simulink subsystem "evitaparedes"  (R2023b)
settings: Solver=VariableStepAuto  StartTime=0.0  StopTime=10.0  RelTol=1e-3
settings Model: Creator=Usuario_UMA  LastModifiedBy=Usuario_UMA

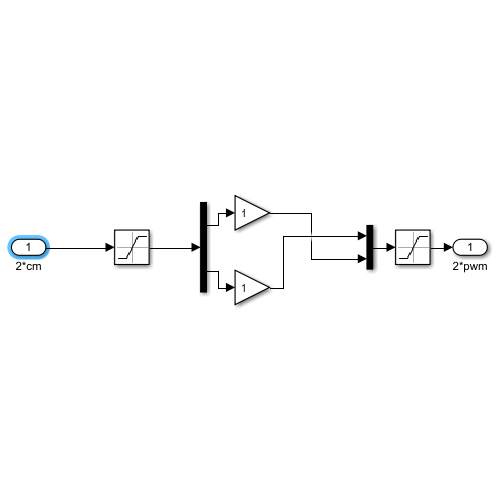
[thumbnail: Simulink's stored preview of the top-level diagram]
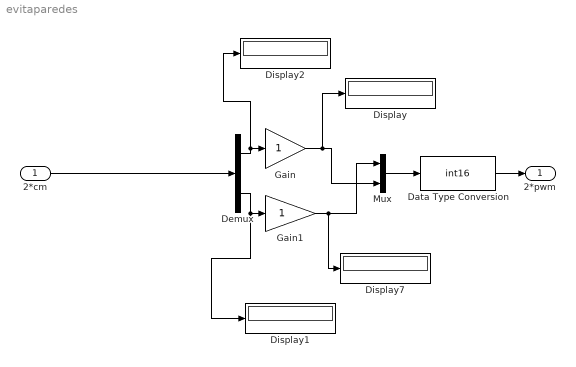
== system evitaparedes ==
  2*cm : Inport
  Data Type Conversion : DataTypeConversion  OutDataTypeStr=int16  SaturateOnIntegerOverflow=off  RndMeth=Floor
  Demux : Demux  Outputs=2
  Display{,1..2,7} (4 alike) : Display
  Gain : Gain
  Gain1 : Gain
  Mux : Mux  Inputs=2
  2*pwm : Outport
  wires:
  Gain/1 -> Mux/2, Display/1
  Mux/1 -> Data Type Conversion/1
  Demux/1 -> Gain/1, Display2/1
  Gain1/1 -> Mux/1, Display7/1
  Demux/2 -> Gain1/1, Display1/1
  2*cm/1 -> Demux/1
  Data Type Conversion/1 -> 2*pwm/1
